simulink model "MPC_constrained"  (R2024b)
settings: Solver=VariableStepAuto  StartTime=0.0  StopTime=tsim  RelTol=1e-3
values from neighbouring files (symbols this model uses):
  C_state = eye(12)    [main.m]
  D_state = zeros(12, 1)    [main.m]
  Q_LQ = q * eye(12)    [main.m]
  R_LQ = r    (= 1e-05)    [main.m]
  S = zeros(n)    [main.m]
  Ts = 0.1    [main.m]    (also in point7.m)
  Ubar_z = inv(dcgain(Gz))*Ybar    [main.m]
  umax = +15    (= 15)    [main.m]
  umin = -15    [main.m]
  x0 = [3,0,3,0,3,0,3,0,3,0,3,0]    [main.m]
  Xbar_z = (eye(12) - Az) \ (Bz * Ubar_z)    [main.m]
undefined symbols (not defined in the file or in its folder): Az, Az_bis, Bz, Bz_bis, Cz, mympc_project
settings Model: Creator=faiol  LastModifiedBy=faiol

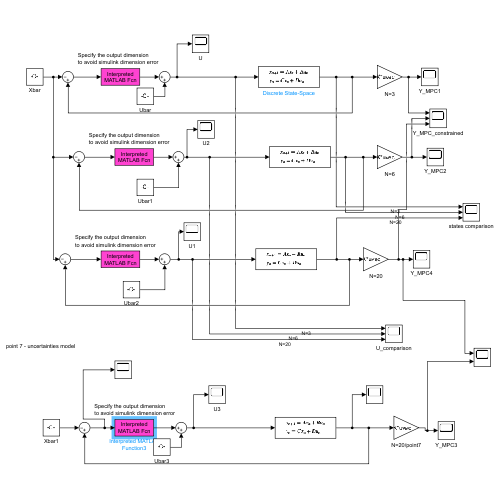
[thumbnail: Simulink's stored preview of the top-level diagram]
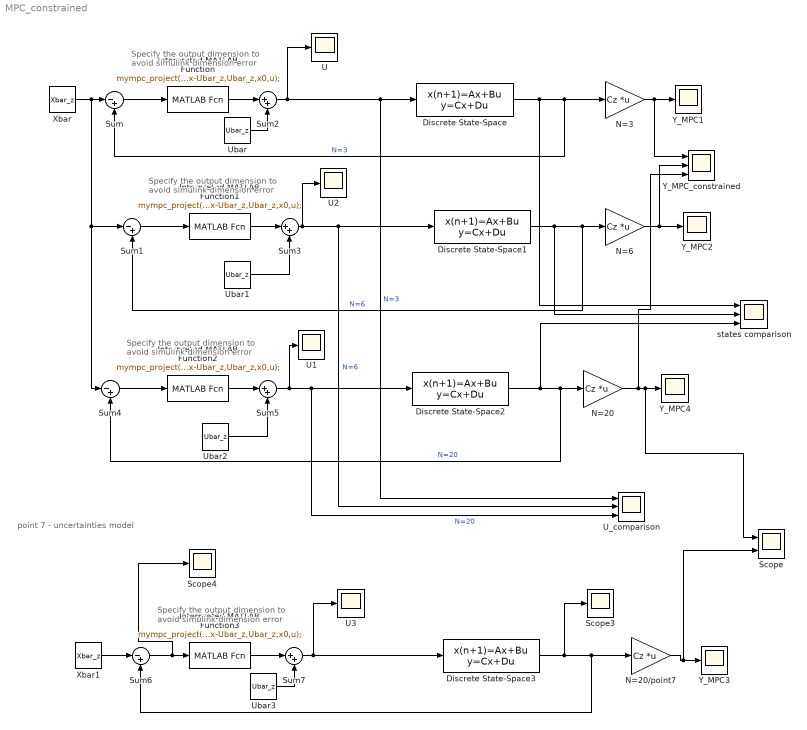
== system MPC_constrained ==
  note: Specify the output dimension
      | to avoid simulink dimension error
  note: Specify the output dimension
      | to avoid simulink dimension error
  note: Specify the output dimension
      | to avoid simulink dimension error
  note: Specify the output dimension
      | to avoid simulink dimension error
  note: point 7 - uncertainties model
  Discrete State-Space : DiscreteStateSpace  A=Az  B=Bz  C=C_state  D=D_state  InitialCondition=x0  SampleTime=Ts
  Discrete State-Space1 : DiscreteStateSpace  A=Az  B=Bz  C=C_state  D=D_state  InitialCondition=x0  SampleTime=Ts
  Discrete State-Space2 : DiscreteStateSpace  A=Az  B=Bz  C=C_state  D=D_state  InitialCondition=x0  SampleTime=Ts
  Discrete State-Space3 : DiscreteStateSpace  A=Az_bis  B=Bz_bis  C=C_state  D=D_state  InitialCondition=x0  SampleTime=Ts
  Interpreted MATLAB Function : MATLABFcn  MATLABFcn=mympc_project(Az,Bz,Q_LQ,R_LQ,S,3,umin-Ubar_z,umax-Ubar_z,Ubar_z,x0,u);  OutputDimensions=1
  Interpreted MATLAB Function1 : MATLABFcn  MATLABFcn=mympc_project(Az,Bz,Q_LQ,R_LQ,S,6,umin-Ubar_z,umax-Ubar_z,Ubar_z,x0,u);  OutputDimensions=1
  Interpreted MATLAB Function2 : MATLABFcn  MATLABFcn=mympc_project(Az,Bz,Q_LQ,R_LQ,S,20,umin-Ubar_z,umax-Ubar_z,Ubar_z,x0,u);  OutputDimensions=1
  Interpreted MATLAB Function3 : MATLABFcn  MATLABFcn=mympc_project(Az,Bz,Q_LQ,R_LQ,S,20,umin-Ubar_z,umax-Ubar_z,Ubar_z,x0,u);  OutputDimensions=1
  N=20 : Gain  Gain=Cz  Multiplication=Matrix(K*u) (u vector)
  N=20/point7 : Gain  Gain=Cz  Multiplication=Matrix(K*u) (u vector)
  N=3 : Gain  Gain=Cz  Multiplication=Matrix(K*u) (u vector)
  N=6 : Gain  Gain=Cz  Multiplication=Matrix(K*u) (u vector)
  Scope : Scope  NumInputPorts=2
  Scope3 : Scope
  Scope4 : Scope
  Sum{,1,4,6} (4 alike) : Sum  Inputs=|-+
  Sum{2..3,5,7} (4 alike) : Sum  Inputs=|++
  U{,1..3} (4 alike) : Scope
  U_comparison : Scope  NumInputPorts=3
  Ubar{,1..3} (4 alike) : Constant  Value=Ubar_z  SampleTime=Ts
  Xbar : Constant  Value=Xbar_z  SampleTime=Ts
  Xbar1 : Constant  Value=Xbar_z  SampleTime=Ts
  Y_MPC{1..4} (4 alike) : Scope
  Y_MPC_constrained : Scope  NumInputPorts=3
  states comparison : Scope  NumInputPorts=3
  wires:
  Discrete State-Space/1 -> states comparison/1, Sum/2, N=3/1  "N=3"
  Xbar/1 -> Sum4/1, Sum1/1, Sum/1
  N=6/1 -> Y_MPC_constrained/2, Y_MPC2/1
  Discrete State-Space1/1 -> states comparison/2, Sum1/2, N=6/1  "N=6"
  Sum3/1 -> U_comparison/2, Discrete State-Space1/1, U2/1  "N=6"
  N=3/1 -> Y_MPC_constrained/1, Y_MPC1/1
  Sum/1 -> Interpreted MATLAB Function/1
  Sum1/1 -> Interpreted MATLAB Function1/1
  Interpreted MATLAB Function/1 -> Sum2/1
  Ubar/1 -> Sum2/2
  Sum2/1 -> U_comparison/1, Discrete State-Space/1, U/1  "N=3"
  Interpreted MATLAB Function1/1 -> Sum3/1
  Ubar1/1 -> Sum3/2
  Interpreted MATLAB Function2/1 -> Sum5/1
  Sum4/1 -> Interpreted MATLAB Function2/1
  Discrete State-Space2/1 -> states comparison/3, Sum4/2, N=20/1  "N=20"
  N=20/1 -> Y_MPC_constrained/3, Scope/1, Y_MPC4/1
  Ubar2/1 -> Sum5/2
  Sum5/1 -> U_comparison/3, Discrete State-Space2/1, U1/1  "N=20"
  Ubar3/1 -> Sum7/2
  N=20/point7/1 -> Scope/2, Y_MPC3/1
  Xbar1/1 -> Sum6/1
  Sum6/1 -> Scope4/1, Interpreted MATLAB Function3/1
  Discrete State-Space3/1 -> Scope3/1, Sum6/2, N=20/point7/1
  Interpreted MATLAB Function3/1 -> Sum7/1
  Sum7/1 -> Discrete State-Space3/1, U3/1
